simulink model "scalar_hw"  (R2023b)
settings: Solver=FixedStepAuto  StartTime=0.0  StopTime=Inf  RelTol=1e-3  EnableMultiTasking=on
values from neighbouring files (symbols this model uses):
  kpp = 3/2 * K^(-2)    (= 1.5)    [init_hw.m]    (also in init_psc_hw.m)
  n = 500    [init_hw.m]    (also in init_psc_hw.m = 300)
  T_pwm = f_clk/(div*f_sw*carr)    (= 9000)    [init_hw.m]    (also in init_psc_hw.m)
  T_s = 1/(2*f_sw)    (= 0.0001)    [init_hw.m]    (also in init_psc_hw.m)
  u_gN = 24    [init_hw.m]    (also in init_psc_hw.m)
  w0_pll = 2*pi*20    (= 125.663706144)    [init_hw.m]    (also in init_psc_hw.m)
  w_b = 0.1*w_N    (= 31.4159265359)    [init_hw.m]    (also in init_psc_hw.m)
  w_N = 2*pi*50    (= 314.159265359)    [init_hw.m]    (also in init_psc_hw.m)
undefined symbols (not defined in the file or in its folder): Down, GPTRIP1SEL, GPTRIP2SEL, TZ1, TZ2, Up
libraries: c2802xlib x13, c2806xlib x4, c280xlib x2, c2000lib x1, simulink x1
(part 1 of 2)
settings Model: SimulationMode=external  ExtModeTrigDuration=15  Creator=maatt  LastModifiedBy=maatt
settings DataIOCC: SaveOutput=off  SignalLogging=off  DSMLogging=off  SaveTime=off  ReturnWorkspaceOutputs=off
settings OptimizationCC: DefaultUnderspecifiedDataType=single  EnhancedBackFolding=on  PassReuseOutputArgsAs=Individual arguments  MaxStackSize=1024  OptimizeBlockOrder=speed  DifferentSizesBufferReuse=on  OptimizationCustomize=off  EfficientTunableParamExpr=on
settings DebuggingCC: ParameterTunabilityLossMsg=error
settings HardwareCC: ProdBitPerChar=16  ProdBitPerInt=16  ProdBitPerPointer=32  ProdBitPerSizeT=32  ProdBitPerPtrDiffT=32  ProdLargestAtomicInteger=Integer  ProdLargestAtomicFloat=None  ProdWordSize=16  ProdLongLongMode=on  ProdHWDeviceType=Texas Instruments->C2000  HardwareBoardFeatureSet=SoCBlockset
settings ModelReferenceCC: ModelReferenceNumInstancesAllowed=Single
settings SFSimCC: MATLABDynamicMemAlloc=off
settings RTWCC: Description=Embedded Coder  SystemTargetFile=ert.tlc  HardwareBoard=TI Piccolo F28069M LaunchPad  TemplateMakefile=ert_default_tmf  Toolchain=Texas Instruments Code Composer Studio (C2000)  CodeProfilingSaveOptions=MetricsOnly
settings CodeAppCC: ForceParamTrailComments=on  IgnoreCustomStorageClasses=off  OperatorAnnotations=on  SimulinkDataObjDesc=on  SFDataObjDesc=on  InsertBlockDesc=on
settings ERTTargetCC: CodeReplacementLibrary=TI C28x  ExtModeTransport=4  ExtModeStaticAlloc=on  ExtModeAutomaticAllocSize=off  ExtModeStaticAllocSize=2000  ExtModeMexFile=ext_xcp  ExtModeIntrfLevel=Level2 - Open

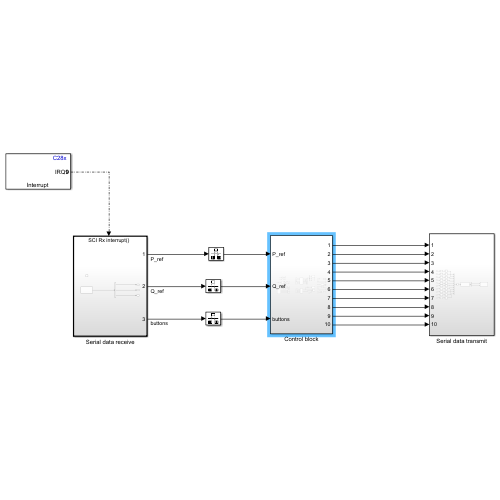
[thumbnail: Simulink's stored preview of the top-level diagram]
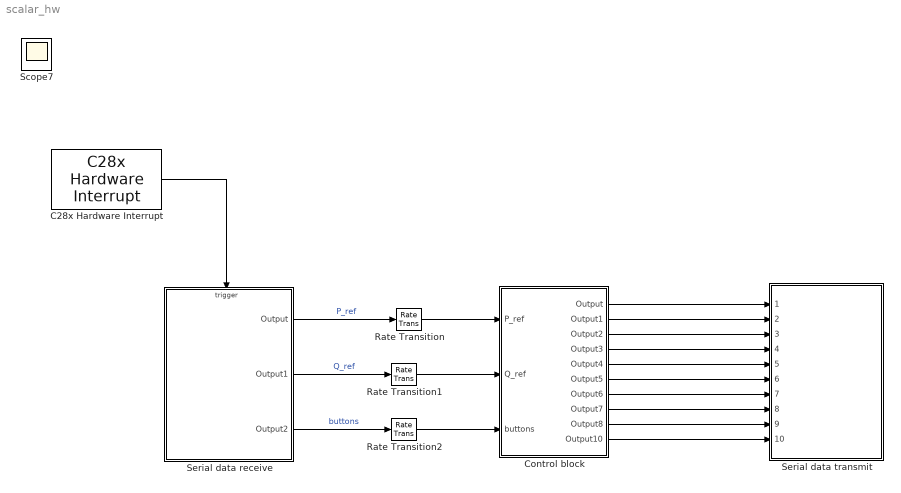
== system scalar_hw ==
  C28x Hardware Interrupt : c2000lib/Scheduling/C28x Hardware Interrupt  irqnumbers=[9]  pienumbers=[1]  irqpriorities=[50]  irqpreempts=[0]  showinput=off  dspchiptype=C280X
  Control block : Subsystem
  Rate Transition : RateTransition  Deterministic=off  OutPortSampleTime=T_s
  Rate Transition1 : RateTransition  Deterministic=off  OutPortSampleTime=T_s
  Rate Transition2 : RateTransition  Deterministic=off  OutPortSampleTime=T_s
  Serial data receive : Subsystem
  Serial data transmit : Subsystem
  Scope7 : Scope
  wires:
  Control block/9(Output8) -> Serial data transmit/9(9)
  Serial data receive/3(Output2) -> Rate Transition2/1  "buttons"
  Control block/5(Output4) -> Serial data transmit/5(5)
  Control block/7(Output6) -> Serial data transmit/7(7)
  Serial data receive/2(Output1) -> Rate Transition1/1  "Q_ref"
  Control block/2(Output1) -> Serial data transmit/2(2)
  Control block/1(Output) -> Serial data transmit/1(1)
  Control block/6(Output5) -> Serial data transmit/6(6)
  Control block/3(Output2) -> Serial data transmit/3(3)
  Control block/4(Output3) -> Serial data transmit/4(4)
  Rate Transition/1 -> Control block/1(P_ref)
  Control block/8(Output7) -> Serial data transmit/8(8)
  Rate Transition1/1 -> Control block/2(Q_ref)
  Control block/10(Output10) -> Serial data transmit/10(10)
  C28x Hardware Interrupt/1 -> Serial data receive/Trigger
  Serial data receive/1(Output) -> Rate Transition/1  "P_ref"
  Rate Transition2/1 -> Control block/3(buttons)

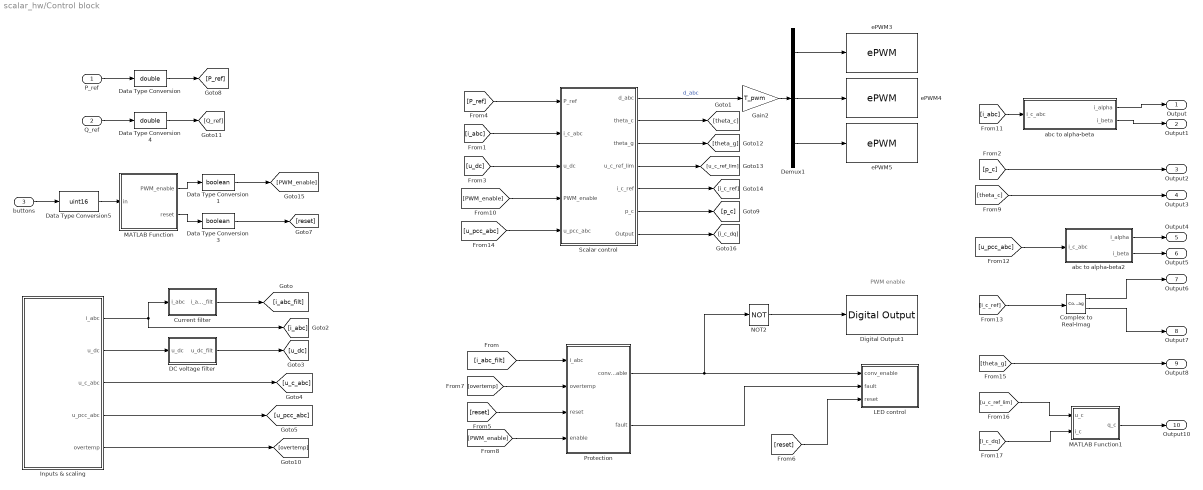
== system scalar_hw/Control block ==
  note: PWM enable
  P_ref : Inport
  Q_ref : Inport  Port=2
  buttons : Inport  Port=3
  Complex to Real-Imag : ComplexToRealImag
  Current filter : Subsystem
  DC voltage filter : Subsystem
  Data Type Conversion : DataTypeConversion  OutDataTypeStr=double  SaturateOnIntegerOverflow=off  RndMeth=Floor
  Data Type Conversion1 : DataTypeConversion  OutDataTypeStr=boolean  SaturateOnIntegerOverflow=off  RndMeth=Floor
  Data Type Conversion3 : DataTypeConversion  OutDataTypeStr=boolean  SaturateOnIntegerOverflow=off  RndMeth=Floor
  Data Type Conversion4 : DataTypeConversion  OutDataTypeStr=double  SaturateOnIntegerOverflow=off  RndMeth=Floor
  Data Type Conversion5 : DataTypeConversion  OutDataTypeStr=uint16  ConvertRealWorld=Stored Integer (SI)  RndMeth=Simplest  SaturateOnIntegerOverflow=off
  Demux1 : Demux  Outputs=3
  Digital Output1 : c2806xlib/Digital Output  GPIO_Number=GPIO50~GPIO55  GPIO_Bit0=off  GPIO_BIT0_Toggle=off  GPIO_Bit1=off  GPIO_BIT1_Toggle=off  GPIO_Bit2=off  GPIO_BIT2_Toggle=off  GPIO_Bit3=off  GPIO_BIT3_Toggle=off  GPIO_Bit4=on  GPIO_BIT4_Toggle=off  GPIO_Bit5=off  GPIO_BIT5_Toggle=off  GPIO_Bit6=off  GPIO_BIT6_Toggle=off  GPIO_Bit7=off  GPIO_BIT7_Toggle=off
  Gain2 : Gain  Gain=T_pwm
  Inputs & scaling : Subsystem
  LED control : Subsystem
  MATLAB Function : MATLAB Function  TreatAsAtomicUnit=on  SystemSampleTime=T_s
  MATLAB Function1 : MATLAB Function  TreatAsAtomicUnit=on  SystemSampleTime=T_s
  NOT2 : Logic  Operator=NOT  IconShape=distinctive  AllPortsSameDT=off  OutDataTypeStr=boolean
  Protection : Subsystem
  Scalar control : Subsystem
  abc to alpha-beta : MATLAB Function  TreatAsAtomicUnit=on  SystemSampleTime=T_s
  abc to alpha-beta2 : MATLAB Function  TreatAsAtomicUnit=on  SystemSampleTime=T_s
  ePWM3 : c2802xlib/ePWM  PwmType=C2000  useModule=ePWM4  ePWMxLINKTBPRD=Not Linked  periodUnits=Clock cycles  timerSource=Specify via dialog  timerPeriod_clk=T_pwm + 1  timerPeriod_sec=0.0001  tbshadow=Counter equals to zero  countingMode=Up-Down  phaseActiveEnable=Disable  phaseDirection=Count down after sync  phaseActive=0  synchronizationEnable=off  dcaevt1Sync=off  dcbevt1Sync=off  synchronizationOption=Counter equals to zero (CTR=Zero)  dcbevt1SyncOut=off  dcaevt1SyncOut=off  cmpdSyncOut=off  cmpcSyncOut=off  cmpbSyncOut=off  zeroSyncOut=off  swfSyncOut=off  perSynchronizationOption=Counter equals to period (CTR=PRD)  clockPrescale=1  HSclockPrescale=1  enswap=off  ePWMxAStatus=on  ePWMxAactionLogic1=Do nothing  ePWMxAactionLogic2=Do nothing  ePWMxAactionLogic3=Clear  ePWMxAactionLogic4=Set  ePWMxAactionLogic5=Do nothing  ePWMxAactionLogic6=Do nothing  ePWMxACSFenable=off  ePWMxACSFvalue=Forcing disable  ePWMxASFreload=Zero  ePWMxBStatus=off  ePWMxBactionLogic1=Set  ePWMxBactionLogic2=Clear  ePWMxBactionLogic3=Do nothing  ePWMxBactionLogic4=Do nothing  ePWMxBactionLogic5=Clear  ePWMxBactionLogic6=Set  ePWMxBCSFenable=off  ePWMxBCSFvalue=Forcing disable  ePWMxBSFreload=Zero  ePWNxBOutWay=off  ePWMxLINKCMPA=Not Linked  CMPAUnits=Clock cycles  CMPASource=Input port  CMPAValue_per=50  CMPAValue_clk=T_pwm/2  enCMPAshadow=Counter equals to zero (CTR=Zero)  ePWMxLINKCMPB=Not Linked  CMPBUnits=Clock cycles  CMPBSource=Specify via dialog  CMPBValue_per=50  CMPBValue_clk=T_pwm/2  enCMPBshadow=Counter equals to zero (CTR=Zero)  ePWMxLINKCMPC=Not Linked  CMPCUnits=Clock cycles  CMPCSource=Specify via dialog  CMPCValue_per=50  CMPCValue_clk=32000  enCMPCshadow=Counter equals to zero (CTR=Zero)  ePWMxLINKCMPD=Not Linked  CMPDUnits=Clock cycles  CMPDSource=Specify via dialog  CMPDValue_per=50  CMPDValue_clk=32000  enCMPDshadow=Counter equals to zero (CTR=Zero)  enableDBePWMxA=on  enableDBePWMxB=on  enhalfcycle=off  DBpolarity=Active high complementary (AHC)  DBedgeDelay=Positive  DBSource_ePWMxA=ePWMxA  DBSource_ePWMxB=ePWMxA  DBPeriodUnits=Clock cycles  DBperiodSource=Specify via dialog  REDperiod=15  FEDperiod=15  REDperiod_sec=0  FEDperiod_sec=0  LoadModeDBRED=Immediate without using shadow  LoadModeDBFED=Immediate without using shadow  adcstartModuleA=on  adcrequestEventA=First event  adcstartEventA=Counter equals to zero or period (CTR=Zero or CTR=PRD)  adcstartEventA_type2=Digital Compare Module A Event 1 start of conversion (DCAEVT1.soc)  adcstartModuleB=off  adcrequestEventB=First event  adcstartEventB=Counter equals to zero (CTR=Zero)  adcstartEventB_type2=Counter equals to zero (CTR=Zero)  intEn=off  intPrd=First event  intSel=Counter equals to zero (CTR=Zero)  intSel_type2=Counter equals to zero (CTR=Zero)  hrpe=off  enHRPWM=off  HRPWM_LoadMode=Counter equals to period (CTR=PRD)  HRPWM_CTLMode=Duty or Period control mode  HRPWM_EDGMode=Both edge  hrpeb=off  enHRPWMB=off  HRPWM_LoadModeB=Counter equals to zero (CTR=ZERO)  HRPWM_CTLModeB=Duty or Period control mode  HRPWM_EDGModeB=Both edge  enHRDBRED=off  enHRDBFED=off  enSFO=on  enautoconv=on  chopperEnable=off  chopperFrequency=1  chopperFirstwidth=1  chopperDuty=12.5%  tripZonesource=Specify via dialog  tzselOSHT1=off  tzselOSHT2=off  tzselOSHT3=off  tzselOSHDCAEV1=off  tzselOSHDCBEV1=off  tzselCBC1=off  tzselCBC2=off  tzselCBC3=off  tzselCBCDCAEV2=off  tzselCBCDCBEV2=off  tzselOSHT4=off  tzselOSHT5=off  tzselOSHT6=off  tzselCBC4=off  tzselCBC5=off  tzselCBC6=off  enTzOstIntr=off  enTzCbcIntr=off  enTzDCAEVT1Intr=off  enTzDCAEVT2Intr=off  enTzDCBEVT1Intr=off  enTzDCBEVT2Intr=off  ePWMxAforced=No action  ePWMxBforced=No action  DCAEVT1forced=No action  DCBEVT1forced=No action  DCAEVT2forced=No action  DCBEVT2forced=No action  dcah=Trip Zone 1 input (TZ1)  dcal=Trip Zone 1 input (TZ1)  dcbh=Trip Zone 1 input (TZ1)  dcbl=Trip Zone 1 input (TZ1)  dcah_type2=GPTRIP1SEL/(TZ1)  dcal_type2=GPTRIP2SEL/(TZ2)  dcbh_type2=GPTRIP1SEL/(TZ1)  dcbl_type2=GPTRIP2SEL/(TZ2)  gendcaevt1=Event disabled  gendcaevt2=Event disabled  gendcbevt1=Event disabled  gendcbevt2=Event disabled  dcaevt1src=DCAEVT1 with sync  dcaevt2src=DCAEVT2 with sync  dcbevt1src=DCBEVT1 with sync  dcbevt2src=DCBEVT2 with sync  pulsesel=Counter equals to zero (CTR=Zero)  blankinv=off  blankoffset=0  blankwidth=0  evsrcsel=Filtered version of DCAEVT1 (DCAEVT1FILT)  encape=off
      settings: LibrarySourceBlock=c2806xlib/ePWM
  ePWM4 : c2802xlib/ePWM  PwmType=C2000  useModule=ePWM5  ePWMxLINKTBPRD=Not Linked  periodUnits=Clock cycles  timerSource=Specify via dialog  timerPeriod_clk=T_pwm + 1  timerPeriod_sec=0.0001  tbshadow=Counter equals to zero  countingMode=Up-Down  phaseActiveEnable=Disable  phaseDirection=Count down after sync  phaseActive=0  synchronizationEnable=off  dcaevt1Sync=off  dcbevt1Sync=off  synchronizationOption=Counter equals to zero (CTR=Zero)  dcbevt1SyncOut=off  dcaevt1SyncOut=off  cmpdSyncOut=off  cmpcSyncOut=off  cmpbSyncOut=off  zeroSyncOut=off  swfSyncOut=off  perSynchronizationOption=Counter equals to period (CTR=PRD)  clockPrescale=1  HSclockPrescale=1  enswap=off  ePWMxAStatus=on  ePWMxAactionLogic1=Do nothing  ePWMxAactionLogic2=Do nothing  ePWMxAactionLogic3=Clear  ePWMxAactionLogic4=Set  ePWMxAactionLogic5=Do nothing  ePWMxAactionLogic6=Do nothing  ePWMxACSFenable=off  ePWMxACSFvalue=Forcing disable  ePWMxASFreload=Zero  ePWMxBStatus=off  ePWMxBactionLogic1=Set  ePWMxBactionLogic2=Clear  ePWMxBactionLogic3=Do nothing  ePWMxBactionLogic4=Do nothing  ePWMxBactionLogic5=Clear  ePWMxBactionLogic6=Set  ePWMxBCSFenable=off  ePWMxBCSFvalue=Forcing disable  ePWMxBSFreload=Zero  ePWNxBOutWay=off  ePWMxLINKCMPA=Not Linked  CMPAUnits=Clock cycles  CMPASource=Input port  CMPAValue_per=50  CMPAValue_clk=T_pwm/2  enCMPAshadow=Counter equals to zero (CTR=Zero)  ePWMxLINKCMPB=Not Linked  CMPBUnits=Clock cycles  CMPBSource=Specify via dialog  CMPBValue_per=50  CMPBValue_clk=T_pwm/2  enCMPBshadow=Counter equals to zero (CTR=Zero)  ePWMxLINKCMPC=Not Linked  CMPCUnits=Clock cycles  CMPCSource=Specify via dialog  CMPCValue_per=50  CMPCValue_clk=32000  enCMPCshadow=Counter equals to zero (CTR=Zero)  ePWMxLINKCMPD=Not Linked  CMPDUnits=Clock cycles  CMPDSource=Specify via dialog  CMPDValue_per=50  CMPDValue_clk=32000  enCMPDshadow=Counter equals to zero (CTR=Zero)  enableDBePWMxA=on  enableDBePWMxB=on  enhalfcycle=off  DBpolarity=Active high complementary (AHC)  DBedgeDelay=Positive  DBSource_ePWMxA=ePWMxA  DBSource_ePWMxB=ePWMxA  DBPeriodUnits=Clock cycles  DBperiodSource=Specify via dialog  REDperiod=15  FEDperiod=15  REDperiod_sec=0  FEDperiod_sec=0  LoadModeDBRED=Immediate without using shadow  LoadModeDBFED=Immediate without using shadow  adcstartModuleA=on  adcrequestEventA=First event  adcstartEventA=Counter equals to zero or period (CTR=Zero or CTR=PRD)  adcstartEventA_type2=Digital Compare Module A Event 1 start of conversion (DCAEVT1.soc)  adcstartModuleB=off  adcrequestEventB=First event  adcstartEventB=Counter equals to zero (CTR=Zero)  adcstartEventB_type2=Counter equals to zero (CTR=Zero)  intEn=off  intPrd=First event  intSel=Counter equals to zero (CTR=Zero)  intSel_type2=Counter equals to zero (CTR=Zero)  hrpe=off  enHRPWM=off  HRPWM_LoadMode=Counter equals to period (CTR=PRD)  HRPWM_CTLMode=Duty or Period control mode  HRPWM_EDGMode=Both edge  hrpeb=off  enHRPWMB=off  HRPWM_LoadModeB=Counter equals to zero (CTR=ZERO)  HRPWM_CTLModeB=Duty or Period control mode  HRPWM_EDGModeB=Both edge  enHRDBRED=off  enHRDBFED=off  enSFO=on  enautoconv=on  chopperEnable=off  chopperFrequency=1  chopperFirstwidth=1  chopperDuty=12.5%  tripZonesource=Specify via dialog  tzselOSHT1=off  tzselOSHT2=off  tzselOSHT3=off  tzselOSHDCAEV1=off  tzselOSHDCBEV1=off  tzselCBC1=off  tzselCBC2=off  tzselCBC3=off  tzselCBCDCAEV2=off  tzselCBCDCBEV2=off  tzselOSHT4=off  tzselOSHT5=off  tzselOSHT6=off  tzselCBC4=off  tzselCBC5=off  tzselCBC6=off  enTzOstIntr=off  enTzCbcIntr=off  enTzDCAEVT1Intr=off  enTzDCAEVT2Intr=off  enTzDCBEVT1Intr=off  enTzDCBEVT2Intr=off  ePWMxAforced=No action  ePWMxBforced=No action  DCAEVT1forced=No action  DCBEVT1forced=No action  DCAEVT2forced=No action  DCBEVT2forced=No action  dcah=Trip Zone 1 input (TZ1)  dcal=Trip Zone 1 input (TZ1)  dcbh=Trip Zone 1 input (TZ1)  dcbl=Trip Zone 1 input (TZ1)  dcah_type2=GPTRIP1SEL/(TZ1)  dcal_type2=GPTRIP2SEL/(TZ2)  dcbh_type2=GPTRIP1SEL/(TZ1)  dcbl_type2=GPTRIP2SEL/(TZ2)  gendcaevt1=Event disabled  gendcaevt2=Event disabled  gendcbevt1=Event disabled  gendcbevt2=Event disabled  dcaevt1src=DCAEVT1 with sync  dcaevt2src=DCAEVT2 with sync  dcbevt1src=DCBEVT1 with sync  dcbevt2src=DCBEVT2 with sync  pulsesel=Counter equals to zero (CTR=Zero)  blankinv=off  blankoffset=0  blankwidth=0  evsrcsel=Filtered version of DCAEVT1 (DCAEVT1FILT)  encape=off
      settings: LibrarySourceBlock=c2806xlib/ePWM
  ePWM5 : c2802xlib/ePWM  PwmType=C2000  useModule=ePWM6  ePWMxLINKTBPRD=Not Linked  periodUnits=Clock cycles  timerSource=Specify via dialog  timerPeriod_clk=T_pwm + 1  timerPeriod_sec=0.0001  tbshadow=Counter equals to zero  countingMode=Up-Down  phaseActiveEnable=Disable  phaseDirection=Count down after sync  phaseActive=0  synchronizationEnable=off  dcaevt1Sync=off  dcbevt1Sync=off  synchronizationOption=Counter equals to zero (CTR=Zero)  dcbevt1SyncOut=off  dcaevt1SyncOut=off  cmpdSyncOut=off  cmpcSyncOut=off  cmpbSyncOut=off  zeroSyncOut=off  swfSyncOut=off  perSynchronizationOption=Counter equals to period (CTR=PRD)  clockPrescale=1  HSclockPrescale=1  enswap=off  ePWMxAStatus=on  ePWMxAactionLogic1=Do nothing  ePWMxAactionLogic2=Do nothing  ePWMxAactionLogic3=Clear  ePWMxAactionLogic4=Set  ePWMxAactionLogic5=Do nothing  ePWMxAactionLogic6=Do nothing  ePWMxACSFenable=off  ePWMxACSFvalue=Forcing disable  ePWMxASFreload=Zero  ePWMxBStatus=off  ePWMxBactionLogic1=Set  ePWMxBactionLogic2=Clear  ePWMxBactionLogic3=Do nothing  ePWMxBactionLogic4=Do nothing  ePWMxBactionLogic5=Clear  ePWMxBactionLogic6=Set  ePWMxBCSFenable=off  ePWMxBCSFvalue=Forcing disable  ePWMxBSFreload=Zero  ePWNxBOutWay=off  ePWMxLINKCMPA=Not Linked  CMPAUnits=Clock cycles  CMPASource=Input port  CMPAValue_per=50  CMPAValue_clk=T_pwm/2  enCMPAshadow=Counter equals to zero (CTR=Zero)  ePWMxLINKCMPB=Not Linked  CMPBUnits=Clock cycles  CMPBSource=Specify via dialog  CMPBValue_per=50  CMPBValue_clk=T_pwm/2  enCMPBshadow=Counter equals to zero (CTR=Zero)  ePWMxLINKCMPC=Not Linked  CMPCUnits=Clock cycles  CMPCSource=Specify via dialog  CMPCValue_per=50  CMPCValue_clk=32000  enCMPCshadow=Counter equals to zero (CTR=Zero)  ePWMxLINKCMPD=Not Linked  CMPDUnits=Clock cycles  CMPDSource=Specify via dialog  CMPDValue_per=50  CMPDValue_clk=32000  enCMPDshadow=Counter equals to zero (CTR=Zero)  enableDBePWMxA=on  enableDBePWMxB=on  enhalfcycle=off  DBpolarity=Active high complementary (AHC)  DBedgeDelay=Positive  DBSource_ePWMxA=ePWMxA  DBSource_ePWMxB=ePWMxA  DBPeriodUnits=Clock cycles  DBperiodSource=Specify via dialog  REDperiod=15  FEDperiod=15  REDperiod_sec=0  FEDperiod_sec=0  LoadModeDBRED=Immediate without using shadow  LoadModeDBFED=Immediate without using shadow  adcstartModuleA=on  adcrequestEventA=First event  adcstartEventA=Counter equals to zero or period (CTR=Zero or CTR=PRD)  adcstartEventA_type2=Digital Compare Module A Event 1 start of conversion (DCAEVT1.soc)  adcstartModuleB=off  adcrequestEventB=First event  adcstartEventB=Counter equals to zero (CTR=Zero)  adcstartEventB_type2=Counter equals to zero (CTR=Zero)  intEn=off  intPrd=First event  intSel=Counter equals to zero (CTR=Zero)  intSel_type2=Counter equals to zero (CTR=Zero)  hrpe=off  enHRPWM=off  HRPWM_LoadMode=Counter equals to period (CTR=PRD)  HRPWM_CTLMode=Duty or Period control mode  HRPWM_EDGMode=Both edge  hrpeb=off  enHRPWMB=off  HRPWM_LoadModeB=Counter equals to zero (CTR=ZERO)  HRPWM_CTLModeB=Duty or Period control mode  HRPWM_EDGModeB=Both edge  enHRDBRED=off  enHRDBFED=off  enSFO=on  enautoconv=on  chopperEnable=off  chopperFrequency=1  chopperFirstwidth=1  chopperDuty=12.5%  tripZonesource=Specify via dialog  tzselOSHT1=off  tzselOSHT2=off  tzselOSHT3=off  tzselOSHDCAEV1=off  tzselOSHDCBEV1=off  tzselCBC1=off  tzselCBC2=off  tzselCBC3=off  tzselCBCDCAEV2=off  tzselCBCDCBEV2=off  tzselOSHT4=off  tzselOSHT5=off  tzselOSHT6=off  tzselCBC4=off  tzselCBC5=off  tzselCBC6=off  enTzOstIntr=off  enTzCbcIntr=off  enTzDCAEVT1Intr=off  enTzDCAEVT2Intr=off  enTzDCBEVT1Intr=off  enTzDCBEVT2Intr=off  ePWMxAforced=No action  ePWMxBforced=No action  DCAEVT1forced=No action  DCBEVT1forced=No action  DCAEVT2forced=No action  DCBEVT2forced=No action  dcah=Trip Zone 1 input (TZ1)  dcal=Trip Zone 1 input (TZ1)  dcbh=Trip Zone 1 input (TZ1)  dcbl=Trip Zone 1 input (TZ1)  dcah_type2=GPTRIP1SEL/(TZ1)  dcal_type2=GPTRIP2SEL/(TZ2)  dcbh_type2=GPTRIP1SEL/(TZ1)  dcbl_type2=GPTRIP2SEL/(TZ2)  gendcaevt1=Event disabled  gendcaevt2=Event disabled  gendcbevt1=Event disabled  gendcbevt2=Event disabled  dcaevt1src=DCAEVT1 with sync  dcaevt2src=DCAEVT2 with sync  dcbevt1src=DCBEVT1 with sync  dcbevt2src=DCBEVT2 with sync  pulsesel=Counter equals to zero (CTR=Zero)  blankinv=off  blankoffset=0  blankwidth=0  evsrcsel=Filtered version of DCAEVT1 (DCAEVT1FILT)  encape=off
      settings: LibrarySourceBlock=c2806xlib/ePWM
  Output : Outport
  Output1 : Outport  Port=2
  Output2 : Outport  Port=3
  Output3 : Outport  Port=4
  Output4 : Outport  Port=5
  Output5 : Outport  Port=6
  Output6 : Outport  Port=7
  Output7 : Outport  Port=8
  Output8 : Outport  Port=9
  Output10 : Outport  Port=10
  wires:
  P_ref/1 -> Data Type Conversion/1
  Demux1/2 -> ePWM4/1
  Gain2/1 -> Demux1/1
  Demux1/3 -> ePWM5/1
  Scalar control/1(d_abc) -> Gain2/1  "d_abc"
  Inputs & scaling/1(i_abc) -> [i_abc], Current filter/1(i_abc)
  Protection/1(conv_enable) -> LED control/1(conv_enable), NOT2/1
  Protection/2(fault) -> LED control/2(fault)
  Current filter/1(i_abc_filt) -> [i_abc_filt]
  [i_abc_filt] -> Protection/1(i_abc)
  Q_ref/1 -> Data Type Conversion4/1
  Scalar control/2(theta_c) -> [theta_c]
  [i_abc] -> Scalar control/2(i_c_abc)
  Inputs & scaling/2(u_dc) -> DC voltage filter/1(u_dc)
  [u_dc] -> Scalar control/3(u_dc)
  Inputs & scaling/3(u_c_abc) -> [u_c_abc]
  Inputs & scaling/4(u_pcc_abc) -> [u_pcc_abc]
  buttons/1 -> Data Type Conversion5/1
  Data Type Conversion/1 -> [P_ref]
  [P_ref] -> Scalar control/1(P_ref)
  [reset] -> Protection/3(reset)
  [reset] -> LED control/3(reset)
  Inputs & scaling/5(overtemp) -> [overtemp]
  [overtemp] -> Protection/2(overtemp)
  [PWM_enable] -> Protection/4(enable)
  abc to alpha-beta2/1(i_alpha) -> Output4/1
  abc to alpha-beta2/2(i_beta) -> Output5/1
  [i_abc] -> abc to alpha-beta/1(i_c_abc)
  [u_pcc_abc] -> abc to alpha-beta2/1(i_c_abc)
  [u_pcc_abc] -> Scalar control/5(u_pcc_abc)
  Scalar control/3(theta_g) -> [theta_g]
  Demux1/1 -> ePWM3/1
  Scalar control/5(i_c_ref) -> [i_c_ref]
  Scalar control/4(u_c_ref_lim) -> [u_c_ref_lim]
  abc to alpha-beta/1(i_alpha) -> Output/1
  abc to alpha-beta/2(i_beta) -> Output1/1
  [p_c] -> Output2/1
  [theta_c] -> Output3/1
  [i_c_ref] -> Complex to Real-Imag/1
  Complex to Real-Imag/1 -> Output6/1
  Complex to Real-Imag/2 -> Output7/1
  [theta_g] -> Output8/1
  MATLAB Function/1(PWM_enable) -> Data Type Conversion1/1
  MATLAB Function/2(reset) -> Data Type Conversion3/1
  Data Type Conversion3/1 -> [reset]
  [PWM_enable] -> Scalar control/4(PWM_enable)
  Data Type Conversion4/1 -> [Q_ref]
  Data Type Conversion1/1 -> [PWM_enable]
  Data Type Conversion5/1 -> MATLAB Function/1(in)
  Scalar control/6(p_c) -> [p_c]
  [i_c_dq] -> MATLAB Function1/2(i_c)
  [u_c_ref_lim] -> MATLAB Function1/1(u_c)
  MATLAB Function1/1(q_c) -> Output10/1
  Scalar control/7(Output) -> [i_c_dq]
  DC voltage filter/1(u_dc_filt) -> [u_dc]
  NOT2/1 -> Digital Output1/1

== system scalar_hw/Serial data receive ==
  SCI Rx interrupt : TriggerPort  TriggerType=function-call  VariantControl=(inherit)  PortDimensions=1
  Demux : Demux  Outputs=3
  SCI Receive : c280xlib/SCI Receive  Priority=2  sciModule=A  dataHead=''  headerCheckMaxCount=16  dataTail=''  dataType=uint8  dataLenOptions=Length via dialog  dataDim=3  maxDataLength=1  initValue=0  errOption=Output the last received value  errValue=0  sampleTime=-1  blockingMode=off  timeOut=inf  outputStatus=off
      settings: LibrarySourceBlock=c2806xlib/SCI Receive
  Output : Outport
  Output1 : Outport  Port=2
  Output2 : Outport  Port=3
  wires:
  Demux/3 -> Output2/1
  Demux/2 -> Output1/1
  Demux/1 -> Output/1
  SCI Receive/1 -> Demux/1

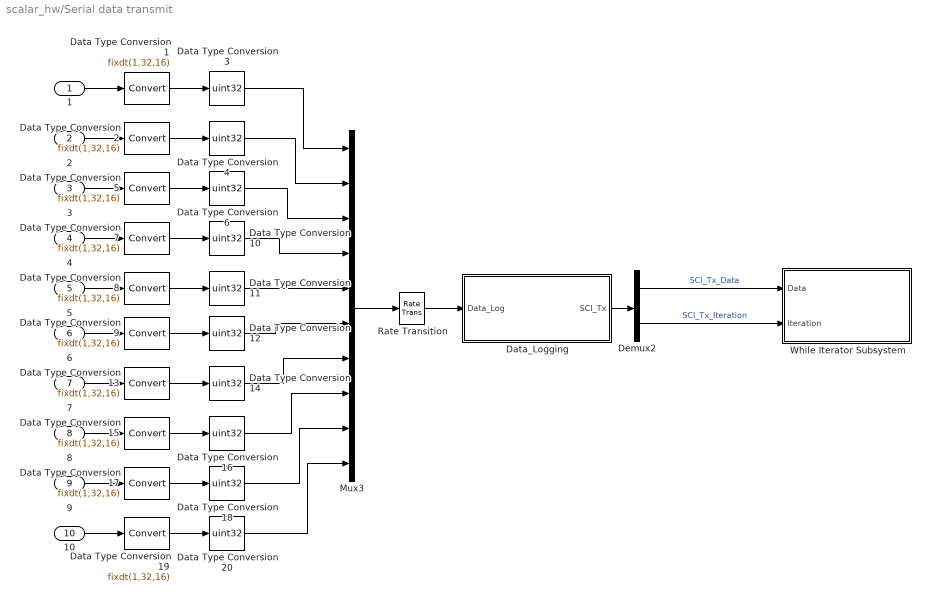
== system scalar_hw/Serial data transmit ==
  1 : Inport
  2 : Inport  Port=2
  3 : Inport  Port=3
  4 : Inport  Port=4
  5 : Inport  Port=5
  6 : Inport  Port=6
  7 : Inport  Port=7
  8 : Inport  Port=8
  9 : Inport  Port=9
  10 : Inport  Port=10
  Data Type Conversion{1..2,5,7..9,13,15,17,19} (10 alike) : DataTypeConversion  OutDataTypeStr=fixdt(1,32,16)  RndMeth=Simplest  SaturateOnIntegerOverflow=off
  Data Type Conversion{3..4,6,10..12,14,16,18,20} (10 alike) : DataTypeConversion  OutDataTypeStr=uint32  ConvertRealWorld=Stored Integer (SI)  RndMeth=Simplest  SaturateOnIntegerOverflow=off
  Data_Logging : Subsystem
  Demux2 : Demux  Outputs=2
  Mux3 : Mux  Inputs=10
  Rate Transition : RateTransition  OutPortSampleTime=4*T_s
  While Iterator Subsystem : Subsystem  TreatAsAtomicUnit=on
  wires:
  Data Type Conversion5/1 -> Data Type Conversion6/1
  7/1 -> Data Type Conversion13/1
  Data_Logging/1(SCI_Tx) -> Demux2/1
  4/1 -> Data Type Conversion7/1
  1/1 -> Data Type Conversion1/1
  Data Type Conversion4/1 -> Mux3/2
  5/1 -> Data Type Conversion8/1
  Data Type Conversion3/1 -> Mux3/1
  2/1 -> Data Type Conversion2/1
  Data Type Conversion8/1 -> Data Type Conversion11/1
  6/1 -> Data Type Conversion9/1
  3/1 -> Data Type Conversion5/1
  Data Type Conversion6/1 -> Mux3/3
  8/1 -> Data Type Conversion15/1
  9/1 -> Data Type Conversion17/1
  10/1 -> Data Type Conversion19/1
  Data Type Conversion1/1 -> Data Type Conversion3/1
  Data Type Conversion2/1 -> Data Type Conversion4/1
  Data Type Conversion7/1 -> Data Type Conversion10/1
  Data Type Conversion9/1 -> Data Type Conversion12/1
  Data Type Conversion13/1 -> Data Type Conversion14/1
  Mux3/1 -> Rate Transition/1
  Data Type Conversion15/1 -> Data Type Conversion16/1
  Data Type Conversion17/1 -> Data Type Conversion18/1
  Data Type Conversion19/1 -> Data Type Conversion20/1
  Data Type Conversion10/1 -> Mux3/4
  Data Type Conversion11/1 -> Mux3/5
  Data Type Conversion12/1 -> Mux3/6
  Data Type Conversion14/1 -> Mux3/7
  Data Type Conversion16/1 -> Mux3/8
  Data Type Conversion18/1 -> Mux3/9
  Data Type Conversion20/1 -> Mux3/10
  Rate Transition/1 -> Data_Logging/1(Data_Log)
  Demux2/1 -> While Iterator Subsystem/1(Data)  "SCI_Tx_Data"
  Demux2/2 -> While Iterator Subsystem/2(Iteration)  "SCI_Tx_Iteration"

== system scalar_hw/Control block/Current filter ==
  i_abc : Inport
  MATLAB Function : MATLAB Function  TreatAsAtomicUnit=on
  Unit Delay : UnitDelay  SampleTime=T_s  HasFrameUpgradeWarning=on
  i_abc_filt : Outport
  wires:
  i_abc/1 -> MATLAB Function/1(i_abc)
  MATLAB Function/1(i_abc_filt_next) -> Unit Delay/1, i_abc_filt/1  "i_filt"
  Unit Delay/1 -> MATLAB Function/2(i_abc_filt)

== system scalar_hw/Control block/DC voltage filter ==
  u_dc : Inport
  MATLAB Function : MATLAB Function  TreatAsAtomicUnit=on
  Unit Delay : UnitDelay  SampleTime=T_s  HasFrameUpgradeWarning=on
  u_dc_filt : Outport
  wires:
  u_dc/1 -> MATLAB Function/1(u_dc)
  MATLAB Function/1(u_dc_filt_next) -> Unit Delay/1, u_dc_filt/1  "i_filt"
  Unit Delay/1 -> MATLAB Function/2(u_dc_filt)

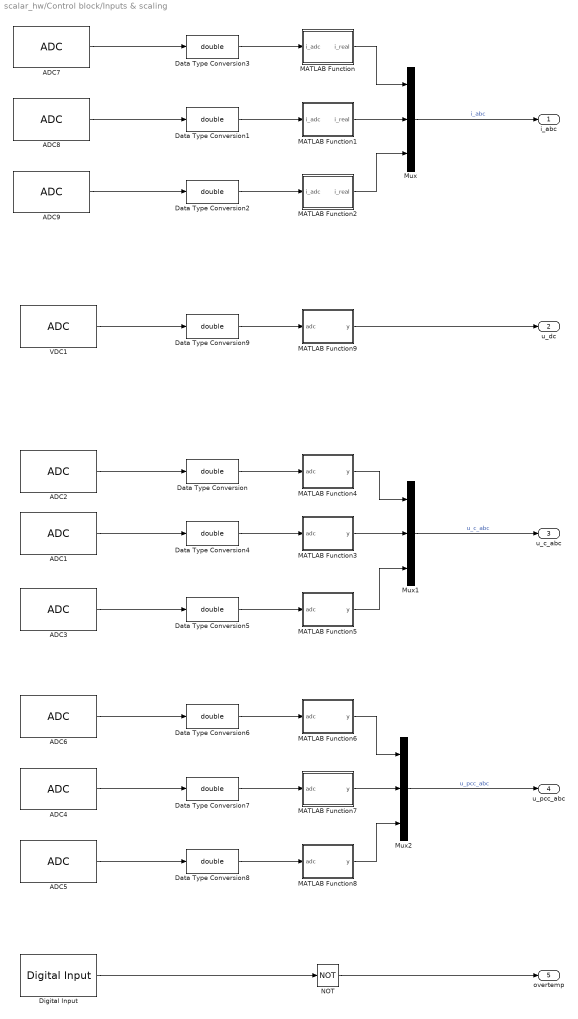
== system scalar_hw/Control block/Inputs & scaling ==
  ADC1 : c2802xlib/ADC  blkParamProc=C2000  ADCModule=1  samplingMode=Single sample mode  ADCResolution=12-bit (Single-ended input)  useSOC1=SOC5  useSOC2=SOC0_SOC1  SOCAcquisitionWindow=15  SOCTriggerSource=ePWM5_ADCSOCA  SOCInterruptTrigger=No ADCINT  Ts=T_s  dType=uint16  postInterrupt=off  interruptSel=ADCINT1  ADCINTContinuous=off  endma=off  chdma=1  conv1=ADCINA5  conv2=ADCINA0 and ADCINB0  conv1_Type4=ADCIN0  conv2_Type4=ADCIN0 and ADCIN1
      settings: LibrarySourceBlock=c2806xlib/ADC
  ADC2 : c2802xlib/ADC  blkParamProc=C2000  ADCModule=1  samplingMode=Single sample mode  ADCResolution=12-bit (Single-ended input)  useSOC1=SOC4  useSOC2=SOC0_SOC1  SOCAcquisitionWindow=15  SOCTriggerSource=ePWM4_ADCSOCA  SOCInterruptTrigger=No ADCINT  Ts=T_s  dType=uint16  postInterrupt=off  interruptSel=ADCINT1  ADCINTContinuous=off  endma=off  chdma=1  conv1=ADCINB4  conv2=ADCINA0 and ADCINB0  conv1_Type4=ADCIN0  conv2_Type4=ADCIN0 and ADCIN1
      settings: LibrarySourceBlock=c2806xlib/ADC
  ADC3 : c2802xlib/ADC  blkParamProc=C2000  ADCModule=1  samplingMode=Single sample mode  ADCResolution=12-bit (Single-ended input)  useSOC1=SOC6  useSOC2=SOC0_SOC1  SOCAcquisitionWindow=15  SOCTriggerSource=ePWM6_ADCSOCA  SOCInterruptTrigger=No ADCINT  Ts=T_s  dType=uint16  postInterrupt=off  interruptSel=ADCINT1  ADCINTContinuous=off  endma=off  chdma=1  conv1=ADCINB5  conv2=ADCINA0 and ADCINB0  conv1_Type4=ADCIN0  conv2_Type4=ADCIN0 and ADCIN1
      settings: LibrarySourceBlock=c2806xlib/ADC
  ADC4 : c2802xlib/ADC  blkParamProc=C2000  ADCModule=1  samplingMode=Single sample mode  ADCResolution=12-bit (Single-ended input)  useSOC1=SOC8  useSOC2=SOC0_SOC1  SOCAcquisitionWindow=15  SOCTriggerSource=ePWM5_ADCSOCA  SOCInterruptTrigger=No ADCINT  Ts=T_s  dType=uint16  postInterrupt=off  interruptSel=ADCINT1  ADCINTContinuous=off  endma=off  chdma=1  conv1=ADCINB1  conv2=ADCINA0 and ADCINB0  conv1_Type4=ADCIN0  conv2_Type4=ADCIN0 and ADCIN1
      settings: LibrarySourceBlock=c2806xlib/ADC
  ADC5 : c2802xlib/ADC  blkParamProc=C2000  ADCModule=1  samplingMode=Single sample mode  ADCResolution=12-bit (Single-ended input)  useSOC1=SOC9  useSOC2=SOC0_SOC1  SOCAcquisitionWindow=15  SOCTriggerSource=ePWM6_ADCSOCA  SOCInterruptTrigger=No ADCINT  Ts=T_s  dType=uint16  postInterrupt=off  interruptSel=ADCINT1  ADCINTContinuous=off  endma=off  chdma=1  conv1=ADCINA2  conv2=ADCINA0 and ADCINB0  conv1_Type4=ADCIN0  conv2_Type4=ADCIN0 and ADCIN1
      settings: LibrarySourceBlock=c2806xlib/ADC
  ADC6 : c2802xlib/ADC  blkParamProc=C2000  ADCModule=1  samplingMode=Single sample mode  ADCResolution=12-bit (Single-ended input)  useSOC1=SOC7  useSOC2=SOC0_SOC1  SOCAcquisitionWindow=15  SOCTriggerSource=ePWM4_ADCSOCA  SOCInterruptTrigger=No ADCINT  Ts=T_s  dType=uint16  postInterrupt=off  interruptSel=ADCINT1  ADCINTContinuous=off  endma=off  chdma=1  conv1=ADCINA7  conv2=ADCINA0 and ADCINB0  conv1_Type4=ADCIN0  conv2_Type4=ADCIN0 and ADCIN1
      settings: LibrarySourceBlock=c2806xlib/ADC
  ADC7 : c2802xlib/ADC  blkParamProc=C2000  ADCModule=1  samplingMode=Single sample mode  ADCResolution=12-bit (Single-ended input)  useSOC1=SOC0  useSOC2=SOC0_SOC1  SOCAcquisitionWindow=15  SOCTriggerSource=ePWM4_ADCSOCA  SOCInterruptTrigger=No ADCINT  Ts=T_s  dType=uint16  postInterrupt=off  interruptSel=ADCINT1  ADCINTContinuous=off  endma=off  chdma=1  conv1=ADCINA3  conv2=ADCINA0 and ADCINB0  conv1_Type4=ADCIN0  conv2_Type4=ADCIN0 and ADCIN1
      settings: LibrarySourceBlock=c2806xlib/ADC
  ADC8 : c2802xlib/ADC  blkParamProc=C2000  ADCModule=1  samplingMode=Single sample mode  ADCResolution=12-bit (Single-ended input)  useSOC1=SOC1  useSOC2=SOC0_SOC1  SOCAcquisitionWindow=15  SOCTriggerSource=ePWM5_ADCSOCA  SOCInterruptTrigger=No ADCINT  Ts=T_s  dType=uint16  postInterrupt=off  interruptSel=ADCINT1  ADCINTContinuous=off  endma=off  chdma=1  conv1=ADCINB3  conv2=ADCINA0 and ADCINB0  conv1_Type4=ADCIN0  conv2_Type4=ADCIN0 and ADCIN1
      settings: LibrarySourceBlock=c2806xlib/ADC
  ADC9 : c2802xlib/ADC  blkParamProc=C2000  ADCModule=1  samplingMode=Single sample mode  ADCResolution=12-bit (Single-ended input)  useSOC1=SOC2  useSOC2=SOC0_SOC1  SOCAcquisitionWindow=15  SOCTriggerSource=ePWM6_ADCSOCA  SOCInterruptTrigger=No ADCINT  Ts=T_s  dType=uint16  postInterrupt=off  interruptSel=ADCINT1  ADCINTContinuous=off  endma=off  chdma=1  conv1=ADCINA4  conv2=ADCINA0 and ADCINB0  conv1_Type4=ADCIN0  conv2_Type4=ADCIN0 and ADCIN1
      settings: LibrarySourceBlock=c2806xlib/ADC
  Data Type Conversion{,1..9} (10 alike) : DataTypeConversion  OutDataTypeStr=double  SaturateOnIntegerOverflow=off  RndMeth=Floor
  Digital Input : c2806xlib/Digital Input  GPIO_Number=GPIO8~GPIO15  GPIO_Bit0=off  GPIO_Bit1=off  GPIO_Bit2=off  GPIO_Bit3=off  GPIO_Bit4=off  GPIO_Bit5=on  GPIO_Bit6=off  GPIO_Bit7=off  sampleTime=T_s  dataType=boolean  GPIO_Bit0_Qualification=Sync to SYSCLKOUT  GPIO_Bit1_Qualification=Sync to SYSCLKOUT  GPIO_Bit2_Qualification=Sync to SYSCLKOUT  GPIO_Bit3_Qualification=Sync to SYSCLKOUT  GPIO_Bit4_Qualification=Sync to SYSCLKOUT  GPIO_Bit5_Qualification=Sync to SYSCLKOUT  GPIO_Bit6_Qualification=Sync to SYSCLKOUT  GPIO_Bit7_Qualification=Sync to SYSCLKOUT  Qualification_Period=-1
  MATLAB Function : MATLAB Function  TreatAsAtomicUnit=on
  MATLAB Function1 : MATLAB Function  TreatAsAtomicUnit=on
  MATLAB Function2 : MATLAB Function  TreatAsAtomicUnit=on
  MATLAB Function3 : MATLAB Function  TreatAsAtomicUnit=on
  MATLAB Function4 : MATLAB Function  TreatAsAtomicUnit=on
  MATLAB Function5 : MATLAB Function  TreatAsAtomicUnit=on
  MATLAB Function6 : MATLAB Function  TreatAsAtomicUnit=on
  MATLAB Function7 : MATLAB Function  TreatAsAtomicUnit=on
  MATLAB Function8 : MATLAB Function  TreatAsAtomicUnit=on
  MATLAB Function9 : MATLAB Function  TreatAsAtomicUnit=on
  Mux : Mux  Inputs=3
  Mux1 : Mux  Inputs=3
  Mux2 : Mux  Inputs=3
  NOT : Logic  Operator=NOT  IconShape=distinctive  AllPortsSameDT=off  OutDataTypeStr=boolean
  VDC1 : c2802xlib/ADC  blkParamProc=C2000  ADCModule=1  samplingMode=Single sample mode  ADCResolution=12-bit (Single-ended input)  useSOC1=SOC3  useSOC2=SOC0_SOC1  SOCAcquisitionWindow=15  SOCTriggerSource=Software  SOCInterruptTrigger=No ADCINT  Ts=T_s  dType=uint16  postInterrupt=off  interruptSel=ADCINT1  ADCINTContinuous=off  endma=off  chdma=1  conv1=ADCINB7  conv2=ADCINA0 and ADCINB0  conv1_Type4=ADCIN0  conv2_Type4=ADCIN0 and ADCIN1
      settings: LibrarySourceBlock=c2806xlib/ADC
  i_abc : Outport
  u_dc : Outport  Port=2
  u_c_abc : Outport  Port=3
  u_pcc_abc : Outport  Port=4
  overtemp : Outport  Port=5
  wires:
  MATLAB Function1/1(i_real) -> Mux/2
  ADC9/1 -> Data Type Conversion2/1
  Data Type Conversion3/1 -> MATLAB Function/1(i_adc)
  MATLAB Function/1(i_real) -> Mux/1
  MATLAB Function2/1(i_real) -> Mux/3
  Data Type Conversion1/1 -> MATLAB Function1/1(i_adc)
  ADC7/1 -> Data Type Conversion3/1
  Data Type Conversion2/1 -> MATLAB Function2/1(i_adc)
  ADC8/1 -> Data Type Conversion1/1
  Mux/1 -> i_abc/1  "i_abc"
  Data Type Conversion/1 -> MATLAB Function4/1(adc)
  Data Type Conversion4/1 -> MATLAB Function3/1(adc)
  Data Type Conversion5/1 -> MATLAB Function5/1(adc)
  Data Type Conversion6/1 -> MATLAB Function6/1(adc)
  Data Type Conversion7/1 -> MATLAB Function7/1(adc)
  Data Type Conversion8/1 -> MATLAB Function8/1(adc)
  ADC5/1 -> Data Type Conversion8/1
  ADC4/1 -> Data Type Conversion7/1
  ADC6/1 -> Data Type Conversion6/1
  ADC3/1 -> Data Type Conversion5/1
  ADC1/1 -> Data Type Conversion4/1
  ADC2/1 -> Data Type Conversion/1
  MATLAB Function4/1(y) -> Mux1/1
  MATLAB Function3/1(y) -> Mux1/2
  MATLAB Function5/1(y) -> Mux1/3
  MATLAB Function6/1(y) -> Mux2/1
  MATLAB Function7/1(y) -> Mux2/2
  MATLAB Function8/1(y) -> Mux2/3
  Mux1/1 -> u_c_abc/1  "u_c_abc"
  Mux2/1 -> u_pcc_abc/1  "u_pcc_abc"
  Data Type Conversion9/1 -> MATLAB Function9/1(adc)
  VDC1/1 -> Data Type Conversion9/1
  MATLAB Function9/1(y) -> u_dc/1
  NOT/1 -> overtemp/1
  Digital Input/1 -> NOT/1

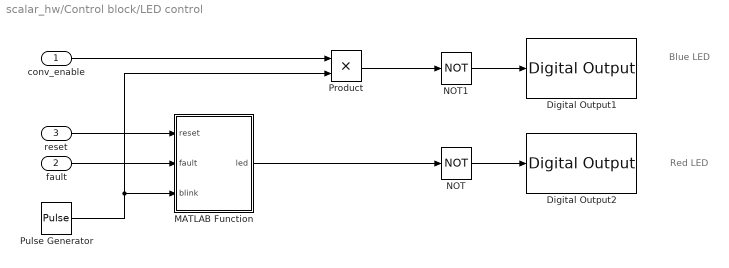
== system scalar_hw/Control block/LED control ==
  note: Blue LED
  note: Red LED
  conv_enable : Inport
  fault : Inport  Port=2
  reset : Inport  Port=3
  Digital Output1 : c2806xlib/Digital Output  GPIO_Number=GPIO32~GPIO39  GPIO_Bit0=off  GPIO_BIT0_Toggle=off  GPIO_Bit1=off  GPIO_BIT1_Toggle=off  GPIO_Bit2=off  GPIO_BIT2_Toggle=off  GPIO_Bit3=off  GPIO_BIT3_Toggle=off  GPIO_Bit4=off  GPIO_BIT4_Toggle=off  GPIO_Bit5=off  GPIO_BIT5_Toggle=off  GPIO_Bit6=off  GPIO_BIT6_Toggle=off  GPIO_Bit7=on  GPIO_BIT7_Toggle=off
  Digital Output2 : c2806xlib/Digital Output  GPIO_Number=GPIO32~GPIO39  GPIO_Bit0=off  GPIO_BIT0_Toggle=off  GPIO_Bit1=off  GPIO_BIT1_Toggle=off  GPIO_Bit2=on  GPIO_BIT2_Toggle=off  GPIO_Bit3=off  GPIO_BIT3_Toggle=off  GPIO_Bit4=off  GPIO_BIT4_Toggle=off  GPIO_Bit5=off  GPIO_BIT5_Toggle=off  GPIO_Bit6=off  GPIO_BIT6_Toggle=off  GPIO_Bit7=off  GPIO_BIT7_Toggle=off
  MATLAB Function : MATLAB Function  TreatAsAtomicUnit=on  SystemSampleTime=T_s
  NOT : Logic  Operator=NOT  IconShape=distinctive  AllPortsSameDT=off  OutDataTypeStr=boolean
  NOT1 : Logic  Operator=NOT  IconShape=distinctive  AllPortsSameDT=off  OutDataTypeStr=boolean
  Product : Product
  Pulse Generator : DiscretePulseGenerator  Period=0.5/T_s  PulseWidth=0.25/T_s  SampleTime=T_s
  wires:
  Pulse Generator/1 -> Product/2, MATLAB Function/3(blink)
  fault/1 -> MATLAB Function/2(fault)
  MATLAB Function/1(led) -> NOT/1
  reset/1 -> MATLAB Function/1(reset)
  Product/1 -> NOT1/1
  conv_enable/1 -> Product/1
  NOT/1 -> Digital Output2/1
  NOT1/1 -> Digital Output1/1

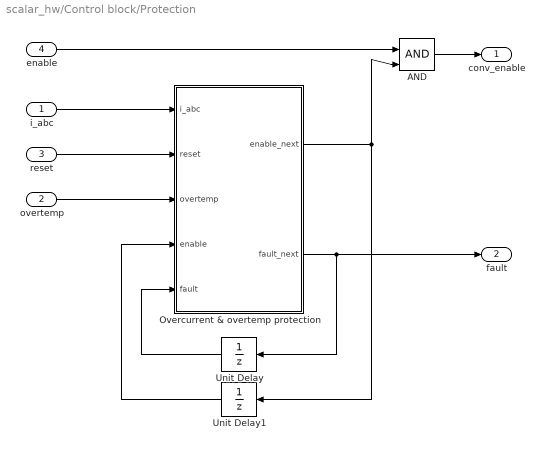
== system scalar_hw/Control block/Protection ==
  i_abc : Inport
  overtemp : Inport  Port=2
  reset : Inport  Port=3
  enable : Inport  Port=4
  AND : Logic  IconShape=distinctive  AllPortsSameDT=off  OutDataTypeStr=boolean
  Overcurrent & overtemp protection : MATLAB Function  TreatAsAtomicUnit=on  SystemSampleTime=T_s
  Unit Delay : UnitDelay  InitialCondition=false  SampleTime=T_s  HasFrameUpgradeWarning=on
  Unit Delay1 : UnitDelay  InitialCondition=false  SampleTime=T_s  HasFrameUpgradeWarning=on
  conv_enable : Outport
  fault : Outport  Port=2
  wires:
  i_abc/1 -> Overcurrent & overtemp protection/1(i_abc)
  reset/1 -> Overcurrent & overtemp protection/2(reset)
  Overcurrent & overtemp protection/1(enable_next) -> AND/2, Unit Delay1/1
  Overcurrent & overtemp protection/2(fault_next) -> fault/1, Unit Delay/1
  Unit Delay1/1 -> Overcurrent & overtemp protection/4(enable)
  Unit Delay/1 -> Overcurrent & overtemp protection/5(fault)
  overtemp/1 -> Overcurrent & overtemp protection/3(overtemp)
  enable/1 -> AND/1
  AND/1 -> conv_enable/1

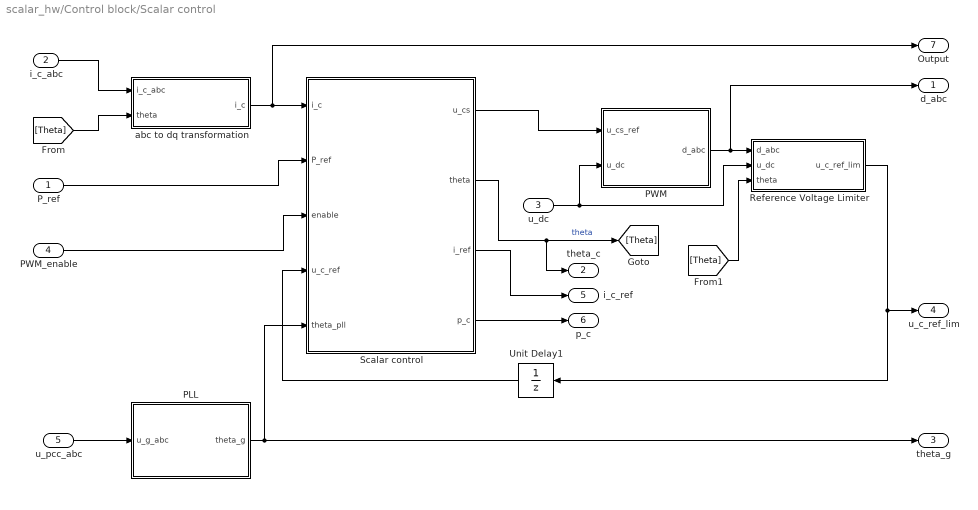
== system scalar_hw/Control block/Scalar control ==
  P_ref : Inport
  i_c_abc : Inport  Port=2
  u_dc : Inport  Port=3
  PWM_enable : Inport  Port=4
  u_pcc_abc : Inport  Port=5
  PLL : Subsystem
  PWM : Subsystem
  Reference Voltage Limiter : Subsystem
  Scalar control : Subsystem
  Unit Delay1 : UnitDelay  SampleTime=T_s  HasFrameUpgradeWarning=on
  abc to dq transformation : MATLAB Function  TreatAsAtomicUnit=on  SystemSampleTime=T_s
  d_abc : Outport
  theta_c : Outport  Port=2
  theta_g : Outport  Port=3
  u_c_ref_lim : Outport  Port=4
  i_c_ref : Outport  Port=5
  p_c : Outport  Port=6
  Output : Outport  Port=7
  wires:
  PWM_enable/1 -> Scalar control/3(enable)
  [Theta] -> Reference Voltage Limiter/3(theta)
  PWM/1(d_abc) -> d_abc/1, Reference Voltage Limiter/1(d_abc)
  Scalar control/1(u_cs) -> PWM/1(u_cs_ref)
  Unit Delay1/1 -> Scalar control/4(u_c_ref)
  P_ref/1 -> Scalar control/2(P_ref)
  abc to dq transformation/1(i_c) -> Output/1, Scalar control/1(i_c)
  u_dc/1 -> Reference Voltage Limiter/2(u_dc), PWM/2(u_dc)
  [Theta] -> abc to dq transformation/2(theta)
  Scalar control/2(theta) -> theta_c/1, [Theta]  "theta"
  i_c_abc/1 -> abc to dq transformation/1(i_c_abc)
  u_pcc_abc/1 -> PLL/1(u_g_abc)
  PLL/1(theta_g) -> Scalar control/5(theta_pll), theta_g/1
  Reference Voltage Limiter/1(u_c_ref_lim) -> u_c_ref_lim/1, Unit Delay1/1
  Scalar control/3(i_ref) -> i_c_ref/1
  Scalar control/4(p_c) -> p_c/1

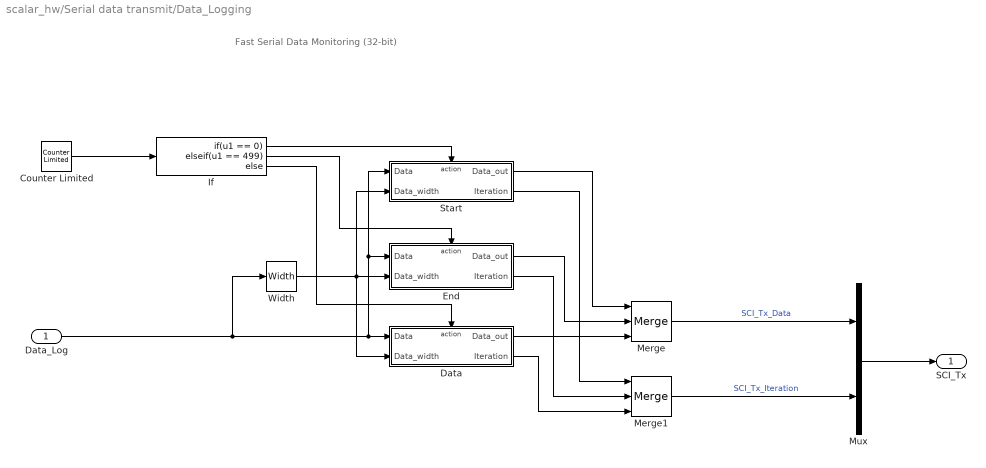
== system scalar_hw/Serial data transmit/Data_Logging ==
  note: Fast Serial Data Monitoring (32-bit)
  Data_Log : Inport
  Counter Limited : simulink/Sources/Counter Limited  uplimit=n-1  tsamp=-1
  Data : Subsystem  TreatAsAtomicUnit=on
  End : Subsystem  TreatAsAtomicUnit=on
  If : If  IfExpression=u1 == 0  ElseIfExpressions=u1 == 499
  Merge : Merge  Inputs=3
  Merge1 : Merge  Inputs=3
  Mux : Mux  Inputs=2
  Start : Subsystem  TreatAsAtomicUnit=on
  Width : Width  OutDataTypeMode=All ports same datatype  DataType=uint16
  SCI_Tx : Outport
  wires:
  If/3 -> Data/Action
  Data/1(Data_out) -> Merge/3
  Width/1 -> Start/2(Data_width), Data/2(Data_width), End/2(Data_width)
  Merge/1 -> Mux/1  "SCI_Tx_Data"
  Counter Limited/1 -> If/1
  Start/2(Iteration) -> Merge1/1
  Start/1(Data_out) -> Merge/1
  If/2 -> End/Action
  Merge1/1 -> Mux/2  "SCI_Tx_Iteration"
  If/1 -> Start/Action
  End/1(Data_out) -> Merge/2
  End/2(Iteration) -> Merge1/2
  Data/2(Iteration) -> Merge1/3
  Mux/1 -> SCI_Tx/1
  Data_Log/1 -> Width/1, Start/1(Data), End/1(Data), Data/1(Data)

== system scalar_hw/Serial data transmit/While Iterator Subsystem ==
  Data : Inport
  Iteration : Inport  Port=2
  Add : Sum  Inputs=+-  OutDataTypeStr=Inherit: Same as first input
  Index Vector : MultiPortSwitch  Inputs=1  SaturateOnIntegerOverflow=off  InputSameDT=off
  SCI Transmit : c280xlib/SCI Transmit  sciModule=A  dataHead=''  dataTail=''  frameSize=1  blockingMode=on  outputStatus=off
  While Iterator : WhileIterator  MaxIters=-1  WhileBlockType=do-while  ShowIterationPort=on  OutputDataType=int16
  wires:
  While Iterator/1 -> Add/2, Index Vector/1
  Data/1 -> Index Vector/2
  Index Vector/1 -> SCI Transmit/1
  Add/1 -> While Iterator/1
  Iteration/1 -> Add/1

== system scalar_hw/Control block/Scalar control/PLL ==
  u_g_abc : Inport
  PLL : MATLAB Function  TreatAsAtomicUnit=on  SystemSampleTime=T_s
  Unit Delay : UnitDelay  InitialCondition=w_N  SampleTime=T_s  HasFrameUpgradeWarning=on
  Unit Delay1 : UnitDelay  SampleTime=T_s  HasFrameUpgradeWarning=on
  theta_g : Outport
  wires:
  u_g_abc/1 -> PLL/1(u_g_abc)
  PLL/2(w_gi_new) -> Unit Delay/1
  PLL/1(theta_g_new) -> Unit Delay1/1
  Unit Delay1/1 -> PLL/2(theta_g), theta_g/1
  Unit Delay/1 -> PLL/3(w_gi)

== system scalar_hw/Control block/Scalar control/PWM ==
  u_cs_ref : Inport
  u_dc : Inport  Port=2
  MATLAB Function : MATLAB Function  TreatAsAtomicUnit=on  SystemSampleTime=T_s
  d_abc : Outport  OutDataTypeStr=double
  wires:
  MATLAB Function/1(d_abc) -> d_abc/1
  u_dc/1 -> MATLAB Function/2(u_dc)
  u_cs_ref/1 -> MATLAB Function/1(u_cs_ref)

== system scalar_hw/Control block/Scalar control/Reference Voltage Limiter ==
  d_abc : Inport
  u_dc : Inport  Port=2
  theta : Inport  Port=3
  MATLAB Function : MATLAB Function  TreatAsAtomicUnit=on  SystemSampleTime=T_s
  u_c_ref_lim : Outport
  wires:
  u_dc/1 -> MATLAB Function/2(u_dc)
  MATLAB Function/1(u_c_ref_lim) -> u_c_ref_lim/1
  theta/1 -> MATLAB Function/3(theta)
  d_abc/1 -> MATLAB Function/1(d_abc)

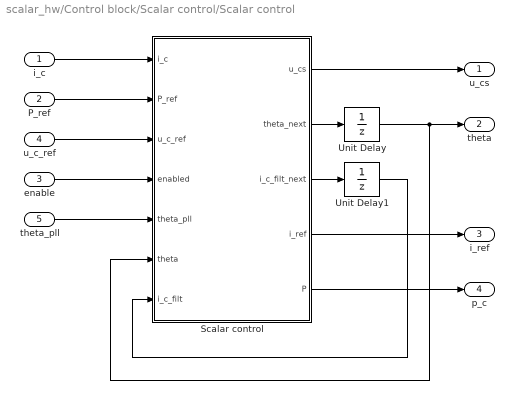
== system scalar_hw/Control block/Scalar control/Scalar control ==
  i_c : Inport
  P_ref : Inport  Port=2
  enable : Inport  Port=3
  u_c_ref : Inport  Port=4
  theta_pll : Inport  Port=5
  Scalar control : MATLAB Function  TreatAsAtomicUnit=on  SystemSampleTime=T_s
  Unit Delay : UnitDelay  SampleTime=T_s  HasFrameUpgradeWarning=on
  Unit Delay1 : UnitDelay  SampleTime=T_s  HasFrameUpgradeWarning=on
  u_cs : Outport  OutDataTypeStr=double
      settings: SignalType=complex
  theta : Outport  Port=2  OutDataTypeStr=double
  i_ref : Outport  Port=3
  p_c : Outport  Port=4
  wires:
  enable/1 -> Scalar control/4(enabled)
  Unit Delay1/1 -> Scalar control/7(i_c_filt)
  Scalar control/3(i_c_filt_next) -> Unit Delay1/1
  Unit Delay/1 -> Scalar control/6(theta), theta/1
  u_c_ref/1 -> Scalar control/3(u_c_ref)
  i_c/1 -> Scalar control/1(i_c)
  P_ref/1 -> Scalar control/2(P_ref)
  Scalar control/2(theta_next) -> Unit Delay/1
  Scalar control/1(u_cs) -> u_cs/1
  theta_pll/1 -> Scalar control/5(theta_pll)
  Scalar control/4(i_ref) -> i_ref/1
  Scalar control/5(P) -> p_c/1

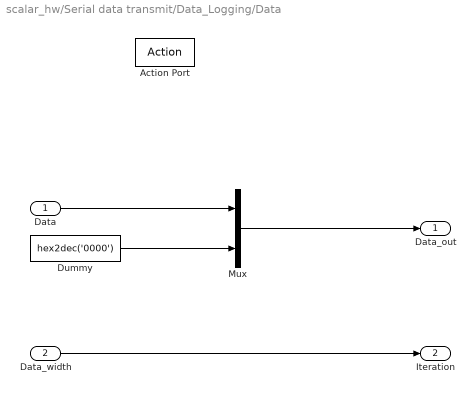
== system scalar_hw/Serial data transmit/Data_Logging/Data ==
  Data : Inport
  Data_width : Inport  Port=2
  Action Port : ActionPort
  Dummy : Constant  Value=hex2dec('0000')  OutDataTypeStr=uint32
  Mux : Mux  Inputs=2
  Data_out : Outport  VectorParamsAs1DForOutWhenUnconnected=off
  Iteration : Outport  Port=2  VectorParamsAs1DForOutWhenUnconnected=off
  wires:
  Data_width/1 -> Iteration/1
  Data/1 -> Mux/1
  Dummy/1 -> Mux/2
  Mux/1 -> Data_out/1

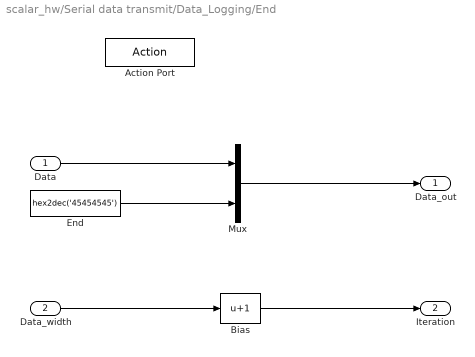
== system scalar_hw/Serial data transmit/Data_Logging/End ==
  Data : Inport
  Data_width : Inport  Port=2
  Action Port : ActionPort
  Bias : Bias  Bias=1  SaturateOnIntegerOverflow=off
  End : Constant  Value=hex2dec('45454545')  OutDataTypeStr=uint32
  Mux : Mux  Inputs=2
  Data_out : Outport  VectorParamsAs1DForOutWhenUnconnected=off
  Iteration : Outport  Port=2  VectorParamsAs1DForOutWhenUnconnected=off
  wires:
  Data/1 -> Mux/1
  Data_width/1 -> Bias/1
  Bias/1 -> Iteration/1
  End/1 -> Mux/2
  Mux/1 -> Data_out/1

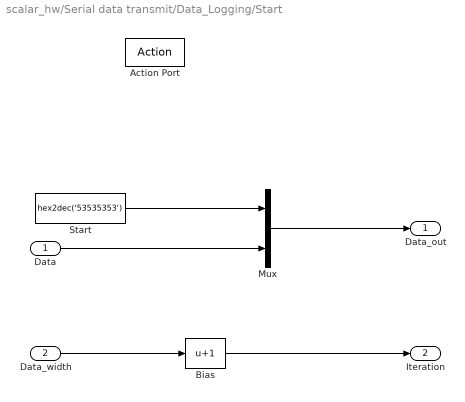
== system scalar_hw/Serial data transmit/Data_Logging/Start ==
  Data : Inport
  Data_width : Inport  Port=2
  Action Port : ActionPort
  Bias : Bias  Bias=1  SaturateOnIntegerOverflow=off
  Mux : Mux  Inputs=2
  Start : Constant  Value=hex2dec('53535353')  OutDataTypeStr=uint32
  Data_out : Outport  VectorParamsAs1DForOutWhenUnconnected=off
  Iteration : Outport  Port=2  VectorParamsAs1DForOutWhenUnconnected=off
  wires:
  Data/1 -> Mux/2
  Data_width/1 -> Bias/1
  Bias/1 -> Iteration/1
  Start/1 -> Mux/1
  Mux/1 -> Data_out/1

== matlab function scalar_hw/Control block/Inputs & scaling/MATLAB Function7 ==
  data: adc input; y output
function y = fcn(adc)

y = (adc*80/4095-4.067)/1.0114 + 5;

== matlab function scalar_hw/Control block/Inputs & scaling/MATLAB Function8 ==
  data: adc input; y output
function y = fcn(adc)

y = (adc*80/4095-4.067)/1.0114 + 5;

== matlab function scalar_hw/Control block/DC voltage filter/MATLAB Function ==
  data: u_dc input double; u_dc_filt_next output double; u_dc_filt input double; w_N parameter; T_s parameter
function u_dc_filt_next = dcvoltagefilter(u_dc, u_dc_filt, w_N, T_s)

w_c=2*pi*w_N;
u_dc_filt_next =  u_dc_filt*(1 - w_c*T_s) + u_dc*(w_c*T_s);

== matlab function scalar_hw/Control block/Protection/Overcurrent & overtemp protection ==
  data: i_abc input double; enable_next output boolean; fault_next output boolean; reset input boolean; overtemp input boolean; enable input boolean; fault input boolean; I_max parameter
function [enable_next, fault_next] = fcn(i_abc, reset, overtemp, enable, fault, I_max)

if(abs(i_abc(1))>=I_max || abs(i_abc(2))>=I_max || abs(i_abc(3))>=I_max)% || overtemp==true)
    fault_state=true;
else
    fault_state=false;
end

if(fault_state==true)
    fault_next=true;
    enable_next=false;
elseif(fault_state==false && reset==true)
    fault_next=false;
    enable_next=true;
else
    fault_next=fault;
    enable_next=enable;
end

== matlab function scalar_hw/Control block/LED control/MATLAB Function ==
  data: reset input boolean; led output; fault input boolean; blink input
function led = fcn(reset, fault, blink)

if(reset==true)
    led=1;
elseif(fault==true)
    led=blink;
else
    led=0;
end

== matlab function scalar_hw/Control block/Current filter/MATLAB Function ==
  data: i_abc input; i_abc_filt_next output; i_abc_filt input; w_N parameter; T_s parameter
function i_abc_filt_next = overcurrentfilter(i_abc, i_abc_filt, w_N, T_s)

w_c=2*pi*w_N;
i_abc_filt_next =  i_abc_filt*(1 - w_c*T_s) + i_abc*(w_c*T_s);

== matlab function scalar_hw/Control block/abc to alpha-beta2 ==
  data: i_alpha output; i_c_abc input; i_beta output
function [i_alpha, i_beta] = fcn(i_c_abc)

% Space Vector Transformation (abc to alpha-beta)
i_cs = 2/3 * (i_c_abc(1) + i_c_abc(2)*exp(1j*2*pi/3) ... 
    + i_c_abc(3)*exp(1j*4*pi/3));

i_alpha = real(i_cs);
i_beta = imag(i_cs);

== matlab function scalar_hw/Control block/Scalar control/PLL/PLL ==
  data: u_g_abc input size=3; theta_g input double; w_gi input double; u_gN parameter; w0_pll parameter; theta_g_new output double; w_gi_new output double; T_s parameter
function [theta_g_new, w_gi_new] = pll(u_g_abc, ...
    theta_g, w_gi, u_gN, w0_pll, T_s)

%theta_g_new = 0;

% Parameters 
% (Tuning of the PLL is analogous to that of the DC-voltage controller.)
zeta = 1;   % Damping ratio
k_p = 2*zeta*w0_pll/u_gN; 
k_i = w0_pll^2/u_gN;

% Space-vector transformation from phase voltages
u_gs = 2/3*(u_g_abc(1) + u_g_abc(2)*exp(1j*2*pi/3) + u_g_abc(3)*exp(1j*4*pi/3));

% Coordinate transformation to the "estimated" grid coordinates
u_g = u_gs*exp(-1j*theta_g);

% Error signal, which is drive to zero by the PLL
u_gq = imag(u_g);

w_g = k_p*u_gq + w_gi;

% Update the integral state
w_gi_new = w_gi + T_s*k_i*u_gq;

% Update the grid-voltage angle
theta_g_new = theta_g + T_s*w_g;
while(theta_g_new > pi)
    theta_g_new = theta_g_new - 2*pi;
end
while(theta_g_new < -pi)
    theta_g_new = theta_g_new + 2*pi;
end

== matlab function scalar_hw/Control block/MATLAB Function ==
  data: in input; PWM_enable output; reset output
function [PWM_enable, reset] = fcn(in)

PWM_enable = bitget(in, 1);
reset = bitget(in, 2);

== matlab function scalar_hw/Control block/Scalar control/Scalar control/Scalar control ==
  data: i_c input; P_ref input; u_cs output double; theta_next output; u_c_ref input; enabled input boolean; theta_pll input; theta input; i_c_filt input; T_s parameter; i_c_filt_next output double; w_b parameter; kpp parameter; w_N parameter; u_gN parameter; i_ref output; P output
function [u_cs, theta_next, i_c_filt_next, i_ref, P] = ... 
    fcn(i_c, P_ref, u_c_ref, enabled, theta_pll, theta, i_c_filt, ... 
    T_s, w_b, kpp, w_N, u_gN)

% Active power calculation
P = 3/2*real(u_c_ref*conj(i_c));

% Equation for grid angular frequency
w_g = w_N;

% Update (integrate) the grid voltage angle
% The converter theta starts uses PLL theta as the starting value when
% enabled (pre-synchronization)
if(enabled==true)
    theta_next = theta + T_s * w_g;
else
     theta_next = theta_pll + T_s * w_g;
end

% Limiting theta to pi >= theta >= -pi
while(theta_next > pi)
    theta_next = theta_next - 2*pi;
end
while(theta_next < -pi)
    theta_next = theta_next + 2*pi;
end

% Extracting the real and imaginary values of the complex converter current
i_c_imag = imag(i_c);

% Applying lowpass filter equation to imaginary part of the
% converter current and forming reference current based on power reference
if(enabled==true)
    i_c_filt_next =  i_c_filt*(1 - w_b*T_s) + i_c_imag*(w_b*T_s);
else
    i_c_filt_next = i_c_filt;
end

% Constructing reference current 
i_ref = P_ref/(u_gN*kpp) + 1j*i_c_filt_next;

% Equation for reference voltage
u_c = u_gN;

% Inverse coordinate transformation
u_cs = u_c*exp(1j*(theta + 1.5 * T_s * w_g));
